simulink model "MPC_paper_Based_Control_1"  (R2025a)
settings: Solver=VariableStepAuto  StartTime=0.0  StopTime=10.0  RelTol=1e-3
libraries: spsCurrentMeasurementLib x4, spsUniversalBridgeLib x4, mpclib x1, eePwmGeneratorMultilevel x1, spsDCVoltageSourceLib x1, spsGroundLib x1, spsSeriesRLCBranchLib x1, sps_lib x1, spsSwitchedReluctanceMotorLib x1
settings Model: Creator=srima  LastModifiedBy=srima

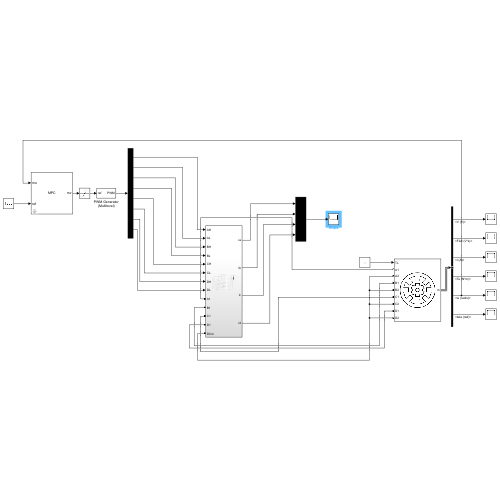
[thumbnail: Simulink's stored preview of the top-level diagram]
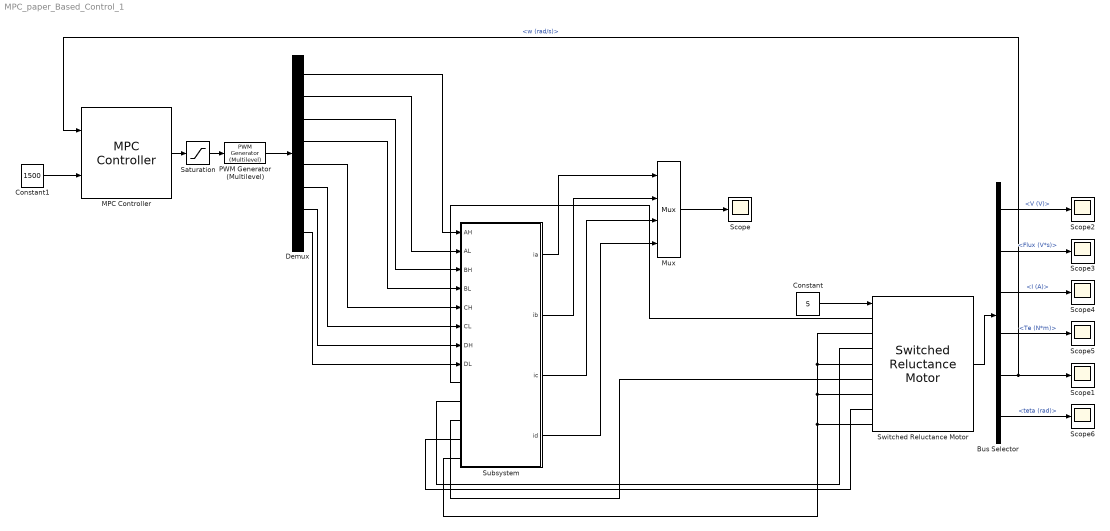
== system MPC_paper_Based_Control_1 ==
  Bus Selector : BusSelector  OutputSignals=V (V),Flux (V*s),I (A),Te (N*m),w (rad/s),teta (rad)
  Constant : Constant  Value=5
  Constant1 : Constant  Value=1500
  Demux : Demux  Outputs=8
  MPC Controller : mpclib/MPC Controller  SCDEnableBlockLinearizationSpecification=on  mpcobj=mpcobj  is_multiple=0  enable_value=0  return_u0=off  updateMPCinCallerWorkspace=on  md_inport=off  mv_inport=off  uref_inport=off  return_cost=off  return_mvseq=off  return_qpstatus=off  return_xseq=off  return_state=off  return_ovseq=off  state_inport=off  umin_inport=off  umax_inport=off  ymin_inport=off  ymax_inport=off  cc_inport=off  ywt_inport=off  uwt_inport=off  duwt_inport=off  rhoeps_inport=off  pm_inport=off  MaximumP=10  HorizonChoice=FixedHorizon  n_ts=0.001  n_p=10  n_mv=1  n_md=1  n_ud=0  n_mo=1  n_uo=0  BlockDataType=double  SampleTimeInherited=off  switch_inport=off
  Mux : Mux
  PWM Generator (Multilevel) : eePwmGeneratorMultilevel/PWM Generator (Multilevel)  topology=Half-bridge  Nsm=4  Tper=0.001  Ts=5e-5
      settings: LibrarySourceBlock=|
      | ee_sl_lib/Pulse Width
      | Modulation/PWM Generator
      | (Multilevel)
  Saturation : Saturate  UpperLimit=0.95  LowerLimit=0
  Scope{,1..6} (7 alike) : Scope
      Scope settings: ActiveDisplayYMinimum=-9392.386561637999  ActiveDisplayYMaximum=84531.479054742013
      Scope1 settings: ActiveDisplayYMinimum=242.82553296717424  ActiveDisplayYMaximum=6764.9467747648014
      Scope2 settings: ActiveDisplayYMinimum=-1801.2382513925927  ActiveDisplayYMaximum=2623.6106321711391  DataLoggingVariableName=ScopeData2
      Scope3 settings: ActiveDisplayYMinimum=-28.299861372487815  ActiveDisplayYMaximum=23.270903541069977  DataLoggingVariableName=ScopeData3
      Scope4 settings: ActiveDisplayYMinimum=-57046.675244211634  ActiveDisplayYMaximum=130016.85043942257  DataLoggingVariableName=ScopeData4
      Scope5 settings: ActiveDisplayYMinimum=27.378762615257358  ActiveDisplayYMaximum=847.19237897659809  DataLoggingVariableName=ScopeData5
      Scope6 settings: ActiveDisplayYMinimum=-133202.42500368995  ActiveDisplayYMaximum=287333.28094710317  DataLoggingVariableName=ScopeData6
  Subsystem : Subsystem
  Switched Reluctance Motor : spsSwitchedReluctanceMotorLib/Switched Reluctance Motor  MachineType=8/6  StatorResistance=0.01  Inertia=0.0082  Friction=0.01  InitialSpeed=[0 0]  TsPowergui=0  TsBlock=-1  MachineModel=Generic model  Lq=0.67e-3  Ld=23.6e-3  Lsat=0.15e-3  MaximumCurrent=450  MaximumFluxLinkage=0.486  Source=MAT-file  MagnetisationCharacteristic='srm64_60kw.mat'  RotorAngleVector=[0 10 20 30 40 45]  StatorCurrentVector=[0:25:450]  PlotCurves=off
      settings: LibrarySourceBlock=|
      | sps_lib/Electrical Machines/Switched Reluctance
      | Motor
  wires:
  Constant/1 -> Switched Reluctance Motor/1
  MPC Controller/1 -> Saturation/1
  Switched Reluctance Motor/1 -> Bus Selector/1
  Bus Selector/5 -> MPC Controller/1, Scope1/1  "<w (rad/s)>"
  Constant1/1 -> MPC Controller/2
  Bus Selector/6 -> Scope6/1  "<teta (rad)>"
  Bus Selector/4 -> Scope5/1  "<Te (N*m)>"
  Bus Selector/3 -> Scope4/1  "<I (A)>"
  Bus Selector/2 -> Scope3/1  "<Flux (V*s)>"
  Bus Selector/1 -> Scope2/1  "<V (V)>"
  Saturation/1 -> PWM Generator (Multilevel)/1
  PWM Generator (Multilevel)/1 -> Demux/1
  Demux/1 -> Subsystem/1(AH)
  Demux/2 -> Subsystem/2(AL)
  Demux/3 -> Subsystem/3(BH)
  Demux/4 -> Subsystem/4(BL)
  Demux/5 -> Subsystem/5(CH)
  Demux/6 -> Subsystem/6(CL)
  Demux/7 -> Subsystem/7(DH)
  Demux/8 -> Subsystem/8(DL)
  Subsystem/1(ia) -> Mux/1
  Subsystem/2(ib) -> Mux/2
  Subsystem/3(ic) -> Mux/3
  Subsystem/4(id) -> Mux/4
  Mux/1 -> Scope/1
  connections:
  Subsystem/LConn1 -- Switched Reluctance Motor/LConn1
  Switched Reluctance Motor/LConn3 -- Subsystem/LConn2
  Subsystem/LConn3 -- Switched Reluctance Motor/LConn5
  Switched Reluctance Motor/LConn7 -- Subsystem/LConn4
  Switched Reluctance Motor/LConn2 -- Subsystem/LConn5 -- Switched Reluctance Motor/LConn8 -- Switched Reluctance Motor/LConn6 -- Switched Reluctance Motor/LConn4

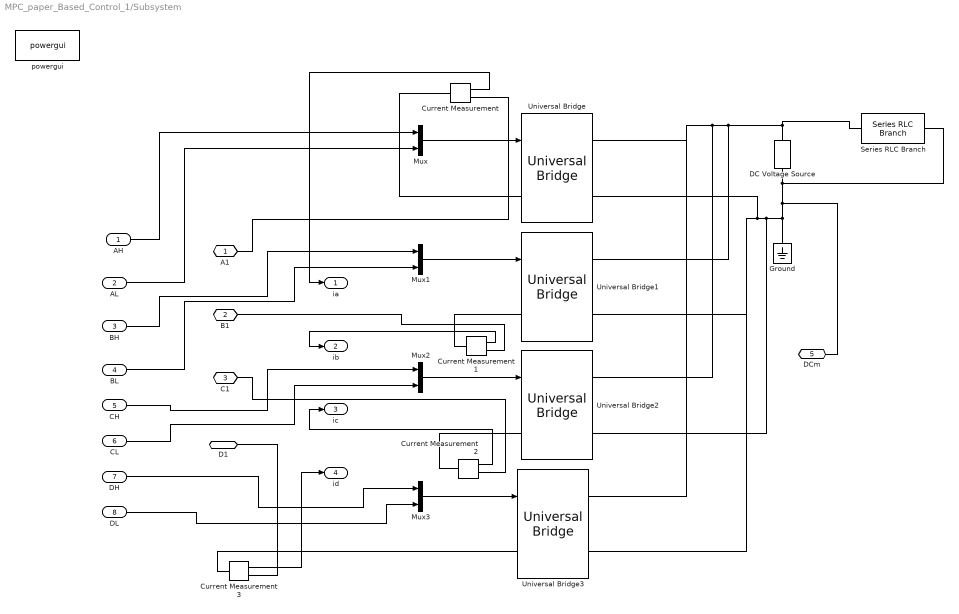
== system MPC_paper_Based_Control_1/Subsystem ==
  AH : Inport
  AL : Inport  Port=2
  BH : Inport  Port=3
  BL : Inport  Port=4
  CH : Inport  Port=5
  CL : Inport  Port=6
  DH : Inport  Port=7
  DL : Inport  Port=8
  Current Measurement{,1..3} (4 alike) : spsCurrentMeasurementLib/Current Measurement  PhasorSimulation=off  OutputType=Complex  PSBequivalent=0
  DC Voltage Source : spsDCVoltageSourceLib/DC Voltage Source  Amplitude=300  Measurements=None
  Ground : spsGroundLib/Ground  LConnTagsString=a
  Mux{,1..3} (4 alike) : Mux  Inputs=2
  Series RLC Branch : spsSeriesRLCBranchLib/Series RLC Branch  LConnTagsString=__new0  RConnTagsString=__new0  BranchType=RC  Resistance=0.5  Inductance=1e-3  SetiL0=off  InitialCurrent=0  Capacitance=2200e-6  Setx0=off  InitialVoltage=0  Measurements=None
  Universal Bridge{,1..3} (4 alike) : spsUniversalBridgeLib/Universal Bridge  Arms=1  SnubberResistance=1e5  SnubberCapacitance=inf  Device=IGBT / Diodes  Ron=1e-3  Lon=0  ForwardVoltages="[  0  0  ]"  ForwardVoltage=0  GTOparameters=[ 10e-6 , 20e-6 ]  IGBTparameters=[ 1e-6 , 2e-6 ]  Measurements=None  Measurements_2=None  converterType=Rectifier
  powergui : sps_lib/powergui  Priority=1  SimulationMode=Discrete  SampleTime=1e-6  frequency=60  Iterations=50  frequencyindice=0  Pbase=100e6  ErrMax=1e-4  UnitsV=kV  UnitsW=MW  buscounter=0  FunctionMessages=off  echomessages=off  EnableUseOfTLC=off  CurrentSourceSwitches=off  DisableSnubberDevices=off  DisableRonSwitches=off  DisableVfSwitches=off  DisplayEquations=off  AutomaticDiscreteSolvers=off  SolverType=Tustin/Backward Euler (TBE)  Interpol=off  ExternalGateDelay=off  methode=off  Ts=100  x0status=blocks  SPID=on  SwTol=0  HookPort=off  NonlinearTolerance=1e-4  nMaxIteration=100  ContinueOnMaxIteration=off  RestoreLinks=warning  ResistiveCurrentMeasurement=off  Frange=[0:2:500]  Ylog=off  Xlog=on  ShowGrid=off  save=off  variable=ZData  structure=0  ZoomFFT=off  StartTime=0.0  cycles=1  DisplayStyle=1  fundamental=60  FreqAxis=off  MaxFrequency=1000  frequencyindicesteady=1  RmsSteady=1  display=off
  A1 : PMIOPort  Side=Left
  B1 : PMIOPort  Port=2  Side=Left
  C1 : PMIOPort  Port=3  Side=Left
  D1 : PMIOPort  Port=4  Side=Left
  DCm : PMIOPort  Port=5  Side=Left
  ia : Outport
  ib : Outport  Port=2
  ic : Outport  Port=3
  id : Outport  Port=4
  wires:
  AH/1 -> Mux/1
  AL/1 -> Mux/2
  Mux/1 -> Universal Bridge/1
  DL/1 -> Mux3/2
  DH/1 -> Mux3/1
  CL/1 -> Mux2/2
  CH/1 -> Mux2/1
  BL/1 -> Mux1/2
  BH/1 -> Mux1/1
  Mux1/1 -> Universal Bridge1/1
  Mux2/1 -> Universal Bridge2/1
  Mux3/1 -> Universal Bridge3/1
  Current Measurement/1 -> ia/1
  Current Measurement1/1 -> ib/1
  Current Measurement2/1 -> ic/1
  Current Measurement3/1 -> id/1
  connections:
  DC Voltage Source/LConn1 -- Series RLC Branch/RConn1 -- DCm/RConn1 -- Universal Bridge2/RConn2 -- Universal Bridge3/RConn2 -- Universal Bridge1/RConn2 -- Universal Bridge/RConn2 -- Ground/LConn1
  Series RLC Branch/LConn1 -- Universal Bridge3/RConn1 -- Universal Bridge/RConn1 -- Universal Bridge2/RConn1 -- Universal Bridge1/RConn1 -- DC Voltage Source/RConn1
  Universal Bridge/LConn1 -- Current Measurement/LConn1
  Universal Bridge2/LConn1 -- Current Measurement2/LConn1
  Universal Bridge3/LConn1 -- Current Measurement3/LConn1
  Universal Bridge1/LConn1 -- Current Measurement1/LConn1
  Current Measurement/RConn1 -- A1/RConn1
  Current Measurement1/RConn1 -- B1/RConn1
  Current Measurement2/RConn1 -- C1/RConn1
  Current Measurement3/RConn1 -- D1/RConn1
